simulink model "sinus"  (Simulink 7.4)
settings: Solver=ode45  StartTime=0.0  StopTime=100  MaxStep=1e-3  RelTol=1e-3
settings Model: Creator=tb42390  LastModifiedBy=fg43085
settings OptimizationCC: InitFltsAndDblsToZero=on
settings DebuggingCC: SaveWithParameterizedLinksMsg=none  SignalResolutionControl=TryResolveAllWithWarning
settings GRTTargetCC: TargetFcnLib=ansi_tfl_tmw.mat

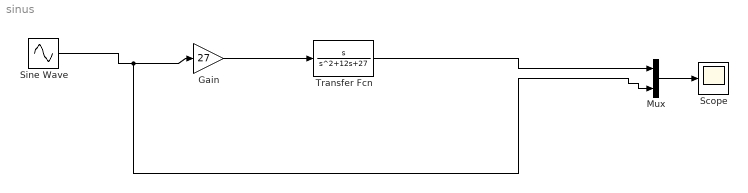
== system sinus ==
  Gain : Gain  Gain=27  ParameterDataType=sfix(16)  ParameterScaling=2^0  OutDataType=sfix(16)  OutScaling=2^0
  Mux : Mux  Inputs=2
  Scope : Scope
      settings: SampleTime=(2*3.14)/4000
  Sine Wave : Sin  Amplitude=1  Bias=0  Frequency=0.1  Phase=0  Samples=10  SampleTime=0  Offset=0
  Transfer Fcn : TransferFcn  Numerator=[1 0]  Denominator=[1 12 27]
  wires:
  Gain/1 -> Transfer Fcn/1
  Sine Wave/1 -> Gain/1, Mux/2
  Transfer Fcn/1 -> Mux/1
  Mux/1 -> Scope/1
